simulink model "SaturationMask"  (R2023a)
settings: Solver=VariableStepAuto  StartTime=0.0  StopTime=10.0  RelTol=1e-3
settings Model: Creator=Egypt_Laptop  LastModifiedBy=Egypt_Laptop

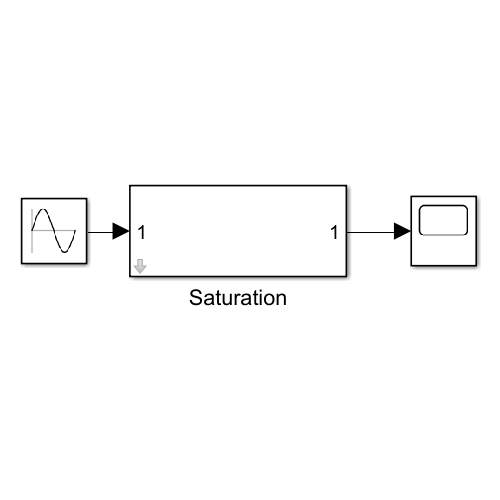
[thumbnail: Simulink's stored preview of the top-level diagram]
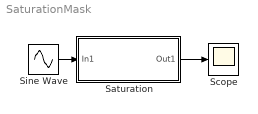
== system SaturationMask ==
  Saturation : Subsystem  mask{UL=0.5, LL=-0.5}
      mask prompts: UL "upperLimit"; LL "LowerLimit"
      mask DialogControl DescGroupVar Prompt: Saturation
  Scope : Scope
  Sine Wave : Sin  SampleTime=0
  wires:
  Sine Wave/1 -> Saturation/1(In1)
  Saturation/1(Out1) -> Scope/1

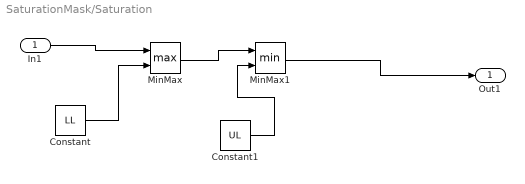
== system SaturationMask/Saturation ==
  In1 : Inport
  Constant : Constant  Value=LL
  Constant1 : Constant  Value=UL
  MinMax : MinMax  Function=max  Inputs=2
  MinMax1 : MinMax  Inputs=2
  Out1 : Outport
  wires:
  In1/1 -> MinMax/1
  Constant/1 -> MinMax/2
  MinMax/1 -> MinMax1/1
  MinMax1/1 -> Out1/1
  Constant1/1 -> MinMax1/2
